simulink model "BeerCupReflexDemo_Spiking"  (R2025a)
settings: Solver=ode45  StartTime=0.0  StopTime=10  RelTol=1e-3
PreLoadFcn:
  | % --- elbow model ---
  | I_el  = 0.06;      % kg*m^2 forearm+cup inertia about elbow
  | b_el  = 2;         % N*m*s/rad damping
  | g     = 9.81;        % m/s^2
  | m_arm = 1.5;         % kg forearm mass
  | Lac   = 0.15;        % m forearm COM distance from elbow
  | Lcup  = 0.3;        % m cup distance from elbow
  | pourRate = 0.0625;   % kg/s beer pour (0.5 kg over 8 s)
  | % --- BPAs (real Festo 20 mm equations) ---
  | Pmax  = 620;         % kPa supply pressure
  | tauAct = 150;      % ms activation
  | L_hold = 0.185;      % m biceps length at level hold
  | c_len = 0.02;      % m biceps length change per rad sag (series compliance)
  | r_bi = 0.04;        % m biceps moment arm
  | L_hold_t = 0.185;   % m triceps length at level hold
  | c_len_t = 0.005;    % m triceps length change per rad sag
  | r_tri = 0.01;       % m triceps moment arm
  | A_bi0 = 0.3923778403;       % biceps activation holding the EMPTY cup (startup equilibrium)
  | A_tri0 = 0.4;      % triceps baseline co-contraction
  | % --- reflex ---
  | desc_bi  = 3.69618892;   % nA descending drive (empty-cup equilibrium)
  | desc_tri = 3.7;  % nA descending drive
  | sagN   = 3.333333333;      % normalize sag rad -> spindle input (~0.3 rad full span)
  | kReflex = 1;         % set 0 in runner to disable reflex synapses
libraries: SNS_Library x20, simulink x1
settings Model: Creator=Ben Bolen  LastModifiedBy=Ben Bolen

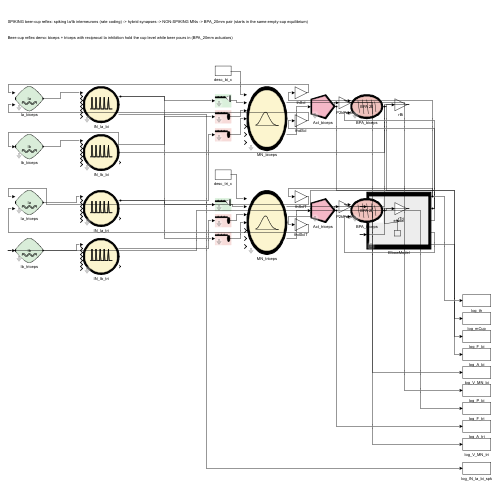
[thumbnail: Simulink's stored preview of the top-level diagram]
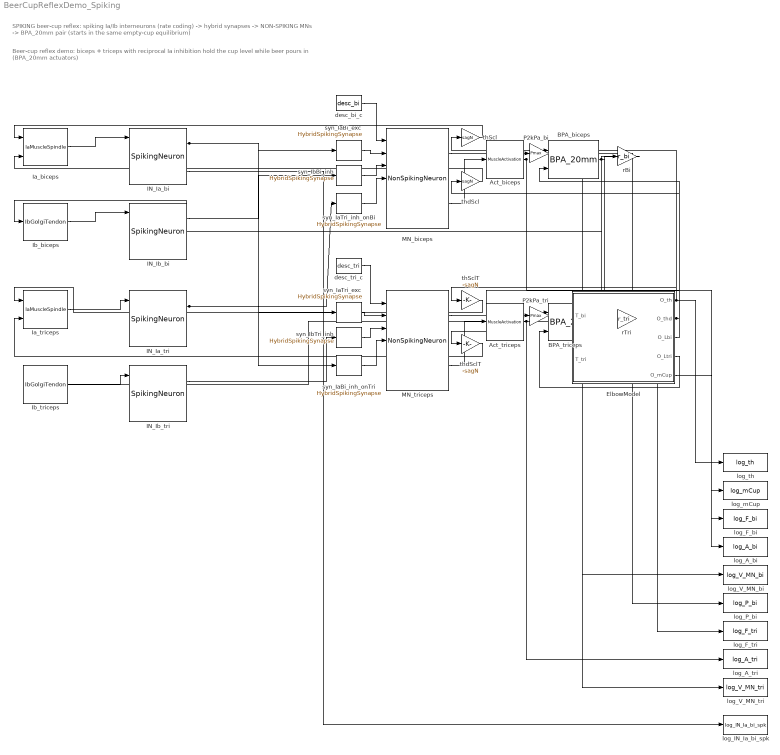
== system BeerCupReflexDemo_Spiking ==
  note: Beer-cup reflex demo: biceps + triceps with reciprocal Ia inhibition hold the cup level while beer pours in (BPA_20mm actuators)
  note: SPIKING beer-cup reflex: spiking Ia/Ib interneurons (rate coding) -> hybrid synapses -> NON-SPIKING MNs -> BPA_20mm pair (starts in the same empty-cup equilibrium)
  Act_biceps : SNS_Library/MuscleActivation  tauAct=tauAct  A0=A_bi0
  Act_triceps : SNS_Library/MuscleActivation  tauAct=tauAct  A0=A_tri0
  BPA_biceps : SNS_Library/BPA_20mm  Rest=0.20  Kmax=0.165  TendonL=0  FittingL=0
  BPA_triceps : SNS_Library/BPA_20mm  Rest=0.20  Kmax=0.165  TendonL=0  FittingL=0
  ElbowModel : Subsystem  mask(SNS Elbow Model (1-DOF)){}
      mask help: 1-DOF elbow with cup: I*thdd = T_biceps - T_triceps - b*thd + T_grav, T_grav = (m_cup(t)*Lcup + m_arm*Lac)*g*cos(theta); beer pours at pourRate. Outputs: theta (sag, rad), thd, biceps length, triceps length, m_cup.
      mask Display:
      | patch([-1 1 1 -1], [-1 -1 1 1], [0 0 0]);
      | patch([-0.92 0.92 0.92 -0.92], [-0.84 -0.84 0.84 0.84], [0.93 0.93 0.93]);
      | color('black');
      | plot([-0.55 -0.45], [0.45 0.45]);
      | plot([-0.45 -0.45], [0.45 -0.10]);
      | plot([-0.45 -0.05], [-0.10 -0.05]);
      | plot([-0.05 -0.05], [-0.05 -0.35]);
      | patch(-0.05 + 0.08*cos(0.3927 + (0:0.0628:1.5708)), -0.05 + 0.08*sin(0.3927 + (0:0.0628:1.5708)), [1 1 1]);
      | patch(-0.05 + 0.05*cos(0.3927 + (0:0.0628:1.5708)), -0.05 + 0.05*sin(0.3927 + (0:0.0628:1.5708)), [0 0 0]);
      | plot([-0.15 0.05 0.05 -0.15 -0.15], [-0.35 -0.35 -0.55 -0.55 -0.35]);
      | disp('elbow');
  IN_Ia_bi : SNS_Library/SpikingNeuron  Vrest=-52  Vth=-46  Vreset=-58  Gm=0.12  Cm=2
  IN_Ia_tri : SNS_Library/SpikingNeuron  Vrest=-52  Vth=-46  Vreset=-58  Gm=0.12  Cm=2
  IN_Ib_bi : SNS_Library/SpikingNeuron  Vrest=-52  Vth=-46  Vreset=-58  Gm=0.4  Cm=2
  IN_Ib_tri : SNS_Library/SpikingNeuron  Vrest=-52  Vth=-46  Vreset=-58  Gm=0.4  Cm=2
  Ia_biceps : SNS_Library/IaMuscleSpindle  Imax=10  Wl=24  Wv=8
  Ia_triceps : SNS_Library/IaMuscleSpindle  Imax=10  Wl=24  Wv=8
  Ib_biceps : SNS_Library/IbGolgiTendon  Imax=10  Kf=0.008
  Ib_triceps : SNS_Library/IbGolgiTendon  Imax=10  Kf=0.008
  MN_biceps : SNS_Library/NonSpikingNeuron  Vrest=-52  Gm=0.5  Cm=5  Thr=-45  Slope=1
  MN_triceps : SNS_Library/NonSpikingNeuron  Vrest=-52  Gm=0.5  Cm=5  Thr=-45  Slope=1
  P2kPa_bi : Gain  Gain=Pmax
  P2kPa_tri : Gain  Gain=Pmax
  desc_bi_c : Constant  Value=desc_bi
  desc_tri_c : Constant  Value=desc_tri
  log_A_bi : ToWorkspace  VariableName=log_A_bi  SaveFormat=Timeseries  SampleTime=-1
  log_A_tri : ToWorkspace  VariableName=log_A_tri  SaveFormat=Timeseries  SampleTime=-1
  log_F_bi : ToWorkspace  VariableName=log_F_bi  SaveFormat=Timeseries  SampleTime=-1
  log_F_tri : ToWorkspace  VariableName=log_F_tri  SaveFormat=Timeseries  SampleTime=-1
  log_IN_Ia_bi_spk : ToWorkspace  VariableName=log_IN_Ia_bi_spk  SaveFormat=Timeseries  SampleTime=-1
  log_P_bi : ToWorkspace  VariableName=log_P_bi  SaveFormat=Timeseries  SampleTime=-1
  log_V_MN_bi : ToWorkspace  VariableName=log_V_MN_bi  SaveFormat=Timeseries  SampleTime=-1
  log_V_MN_tri : ToWorkspace  VariableName=log_V_MN_tri  SaveFormat=Timeseries  SampleTime=-1
  log_mCup : ToWorkspace  VariableName=log_mCup  SaveFormat=Timeseries  SampleTime=-1
  log_th : ToWorkspace  VariableName=log_th  SaveFormat=Timeseries  SampleTime=-1
  rBi : Gain  Gain=r_bi
  rTri : Gain  Gain=r_tri
  syn_IaBi_exc : SNS_Library/HybridSpikingSynapse  gmax=0.01  ginc=0.00057*kReflex  tau_syn=10  Esyn=0  ThrPre=-47
  syn_IaBi_inh_onTri : SNS_Library/HybridSpikingSynapse  gmax=0.01  ginc=0.00285*kReflex  tau_syn=10  Esyn=-72  ThrPre=-47
  syn_IaTri_exc : SNS_Library/HybridSpikingSynapse  gmax=0.01  ginc=0.00114*kReflex  tau_syn=10  Esyn=0  ThrPre=-47
  syn_IaTri_inh_onBi : SNS_Library/HybridSpikingSynapse  gmax=0.01  ginc=0.00091*kReflex  tau_syn=10  Esyn=-72  ThrPre=-47
  syn_IbBi_inh : SNS_Library/HybridSpikingSynapse  gmax=0.01  ginc=0.00068*kReflex  tau_syn=10  Esyn=-72  ThrPre=-47
  syn_IbTri_inh : SNS_Library/HybridSpikingSynapse  gmax=0.01  ginc=0.00046*kReflex  tau_syn=10  Esyn=-72  ThrPre=-47
  thScl : Gain  Gain=sagN
  thSclT : Gain  Gain=-sagN
  thdScl : Gain  Gain=sagN
  thdSclT : Gain  Gain=-sagN
  wires:
  ElbowModel/1(O_th) -> thScl/1, thSclT/1, log_th/1
  ElbowModel/2(O_thd) -> thdScl/1, thdSclT/1
  thScl/1 -> Ia_biceps/1
  thdScl/1 -> Ia_biceps/2
  thSclT/1 -> Ia_triceps/1
  thdSclT/1 -> Ia_triceps/2
  desc_bi_c/1 -> MN_biceps/1
  desc_tri_c/1 -> MN_triceps/1
  MN_biceps/2 -> Act_biceps/1
  MN_triceps/2 -> Act_triceps/1
  Act_biceps/1 -> P2kPa_bi/1, log_A_bi/1
  Act_triceps/1 -> P2kPa_tri/1, log_A_tri/1
  P2kPa_bi/1 -> BPA_biceps/1, log_P_bi/1
  P2kPa_tri/1 -> BPA_triceps/1
  ElbowModel/3(O_Lbi) -> BPA_biceps/2
  ElbowModel/4(O_Ltri) -> BPA_triceps/2
  BPA_biceps/1 -> rBi/1, Ib_biceps/1, log_F_bi/1
  BPA_triceps/1 -> rTri/1, Ib_triceps/1, log_F_tri/1
  rBi/1 -> ElbowModel/1(T_bi)
  rTri/1 -> ElbowModel/2(T_tri)
  ElbowModel/5(O_mCup) -> log_mCup/1
  MN_biceps/1 -> log_V_MN_bi/1
  MN_triceps/1 -> log_V_MN_tri/1
  Ia_biceps/1 -> IN_Ia_bi/1
  Ib_biceps/1 -> IN_Ib_bi/1
  Ia_triceps/1 -> IN_Ia_tri/1
  Ib_triceps/1 -> IN_Ib_tri/1
  IN_Ia_bi/1 -> syn_IaBi_exc/1, syn_IaBi_inh_onTri/1
  IN_Ib_bi/1 -> syn_IbBi_inh/1
  IN_Ia_tri/1 -> syn_IaTri_inh_onBi/1, syn_IaTri_exc/1
  IN_Ib_tri/1 -> syn_IbTri_inh/1
  syn_IaBi_exc/1 -> MN_biceps/2
  syn_IbBi_inh/1 -> MN_biceps/3
  syn_IaTri_inh_onBi/1 -> MN_biceps/4
  syn_IaTri_exc/1 -> MN_triceps/2
  syn_IbTri_inh/1 -> MN_triceps/3
  syn_IaBi_inh_onTri/1 -> MN_triceps/4
  IN_Ia_bi/2 -> log_IN_Ia_bi_spk/1

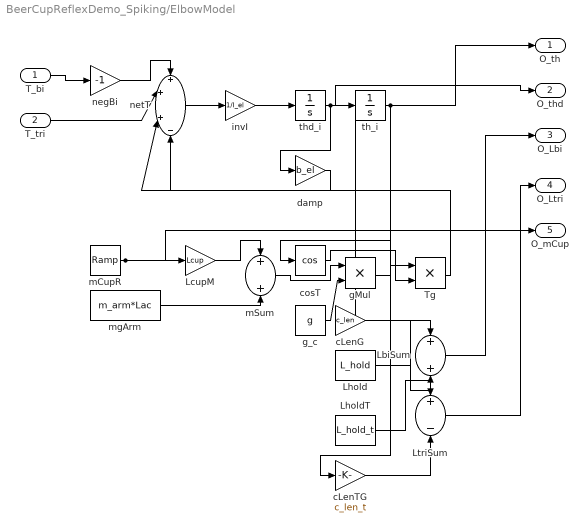
== system BeerCupReflexDemo_Spiking/ElbowModel ==
  T_bi : Inport
  T_tri : Inport  Port=2
  LbiSum : Sum
  LcupM : Gain  Gain=Lcup
  Lhold : Constant  Value=L_hold
  LholdT : Constant  Value=L_hold_t
  LtriSum : Sum  Inputs=+-
  Tg : Product
  cLenG : Gain  Gain=c_len
  cLenTG : Gain  Gain=c_len_t
  cosT : Trigonometry  Operator=cos
  damp : Gain  Gain=b_el
  gMul : Product
  g_c : Constant  Value=g
  invI : Gain  Gain=1/I_el
  mCupR : simulink/Sources/Ramp  slope=pourRate  start=0  InitialOutput=0
  mSum : Sum
  mgArm : Constant  Value=m_arm*Lac
  negBi : Gain  Gain=-1
  netT : Sum  Inputs=+++-
  th_i : Integrator
  thd_i : Integrator
  O_th : Outport
  O_thd : Outport  Port=2
  O_Lbi : Outport  Port=3
  O_Ltri : Outport  Port=4
  O_mCup : Outport  Port=5
  wires:
  T_bi/1 -> negBi/1
  T_tri/1 -> netT/2
  negBi/1 -> netT/1
  netT/1 -> invI/1
  invI/1 -> thd_i/1
  thd_i/1 -> th_i/1, damp/1, O_thd/1
  damp/1 -> netT/4
  th_i/1 -> cosT/1, O_th/1, cLenG/1, cLenTG/1
  mCupR/1 -> LcupM/1, O_mCup/1
  LcupM/1 -> mSum/1
  mgArm/1 -> mSum/2
  mSum/1 -> gMul/1
  g_c/1 -> gMul/2
  gMul/1 -> Tg/1
  cosT/1 -> Tg/2
  Tg/1 -> netT/3
  Lhold/1 -> LbiSum/1
  cLenG/1 -> LbiSum/2
  LbiSum/1 -> O_Lbi/1
  LholdT/1 -> LtriSum/1
  cLenTG/1 -> LtriSum/2
  LtriSum/1 -> O_Ltri/1
